simulink model "WaterRunner_closed3"  (R2013a)
settings: Solver=ode23s  StartTime=0.0  StopTime=10  RelTol=1e-3
values from neighbouring files (symbols this model uses):
  Ac = [sum(Ay), sum(Ath), sum(Aph) ... (first row only)    [SimParam_hopper.m]    (also in simParam.m = [2*sum(Ay), 2*sum(Ath))
  Cgain = 0    [searchHeightWaves.m]    (also in searchTorques.m; simParam.m = 10)
  dTorqueAmp = 1e-2    (= 0.01)    [SimParam_hopper.m]    (also in simParam.m = 0)
  dTorqueFreq = 0.5    [SimParam_hopper.m]    (also in simParam.m = 3.14159265359)
  dWaveAmp = 0    [simParam.m]
  dWaveFreq = (2*pi)/2    (= 3.14159265359)    [simParam.m]
  Filter_Coef = 1000    [SimParam_hopper.m]    (also in simParam.m)
  freq = findSSinput(y,b_water,k_water,A,Fratio,mass*g/4,w0)    [SimParam_hopper.m]    (also in findParams.m = freqs(k); simParam.m; sweepDFomega.m = FREQ(k))
  Gc = [sum(G) - mass*g ; Lx'*G ; Lz'*G]    [SimParam_hopper.m]    (also in simParam.m = [2*sum(G) - mass*g ; Lx'*G ])
  Kdf = 0.25    [SimParam_hopper.m]    (also in simParam.m = 0)
  Ke = diag([0 1])    [simParam.m]
  Mc = [mass 0 0; 0 Ix 0 ; 0 0 Iz]    [SimParam_hopper.m]    (also in simParam.m = [mass 0 ; 0 Ix])
  nullProj = eye(8) - pinvBc*Bc    [SimParam_hopper.m]    (also in simParam.m = eye(4) - pinvBc*Bc)
  omega_0 = freq*ones(8,1)    [SimParam_hopper.m]    (also in findParams.m = freq*ones(4,1); simParam.m = freq*ones(4,1); sweepDFomega.m = freq*ones(4,1))
  phase_0 = [0 pi 0 pi]    [findParams.m]    (also in simParam.m; sweepDFomega.m)
  pinvBc = pinv(Bc)    [SimParam_hopper.m]    (also in simParam.m)
  tail_density = CF_density    (= 1790)    [simParam.m]
  tail_length = 0.1    [simParam.m]
  theta = 0 *pi/180    (= 0)    [SimParam_hopper.m]    (also in simParam.m)
  y = 0.02    [SimParam_hopper.m]    (also in simParam.m = 0.015)
undefined symbols (not defined in the file or in its folder): X, Y, Z
undefined symbols (not defined in the file): cw_FL_HL, cw_FR_FL, cw_FR_HR, cw_HR_HL, FL_HL_lag, FR_FL_lag, FR_HR_lag, HR_HL_lag, K_d, K_i, K_p, phi0, tail_pad_radius, theta0, water_level, y0
libraries: nesl_utility x40, sm_lib x36, WaterRunner_lib_2 x10, dspstat3 x4, simulink x3
(part 1 of 4)
settings Model: SimulationMode=rapid-accelerator  ExtModeTrigDuration=100  Creator=nitisht  LastModifiedBy=nitisht
settings SolverCC: ZeroCrossControl=DisableAll  ZeroCrossAlgorithm=Adaptive
settings DataIOCC: SaveFinalState=on  SignalLoggingSaveFormat=ModelDataLogs  SaveOutput=off  SaveState=on  StateSaveName=tmp_raccel_xout
settings OptimizationCC: BlockReduction=off  ExpressionDepthLimit=2147483647  EfficientMapNaN2IntZero=off  SimCompilerOptimization=On
settings DebuggingCC: SolverPrmCheckMsg=none  FcnCallInpInsideContextMsg=EnableAllAsWarning
settings HardwareCC: ProdBitPerLong=64  ProdBitPerPointer=64  ProdIntDivRoundTo=Zero  ProdEndianess=LittleEndian  ProdWordSize=64  ProdHWDeviceType=Intel->x86-64  TargetBitPerLong=64  TargetBitPerPointer=64  TargetIntDivRoundTo=Zero  TargetEndianess=LittleEndian  TargetWordSize=64  TargetHWDeviceType=MATLAB Host  ProdEqTarget=off
settings RTWCC: SystemTargetFile=raccel.tlc  TemplateMakefile=raccel_default_tmf  RTWVerbose=off  ProcessScript=raccel_make_rtw_hook  RTWUseSimCustomCode=on
settings CodeAppCC: GenerateComments=off  MaxIdLength=128  MangleLength=10  SimulinkBlockComments=off
settings RaccelTargetCC: CodeReplacementLibrary=ANSI_C  ERTMultiwordTypeDef=System defined  ERTMultiwordLength=256  IsPILTarget=off  ParMdlRefBuildCompliant=off  GeneratePreprocessorConditionals=Disable all  ERTFirstTimeCompliant=off  MultiInstanceERTCode=off  EnableShiftOperators=on  ExtModeMexArgs='', 0, 36789  ENABLE_SLEXEC_SSBRIDGE=off  RTWCAPISignals=off  RTWCAPIParams=off
settings ExplorerConfigSet: InternalSimMechanicsExplorerSettings="<ExplorerConfiguration><canonicalview>default</canonicalview><TilePanel><TileInfo><Tiles Columns=\"1\" Count=\"1\" Rows=\"1\"><Column Left=\"2\" Weight=\"1\"/><Column Left=\"1126\"/><Row Top=\"2\" Weight=\"1\"/><Row Top=\"731\"/><Tile Height=\"1\" Width=\"1\" X=\"0\" Y=\"0\"/></Tiles></TileInfo><SceneInfo><SceneViewer><BGColor><R>0.60000002384185791</R><G>0.60000002384185791</G><B>0.60000002384185791</B></BGColor><Camera><Position><X>0.62960776240868022</X><Y>0.44895086159575193</Y><Z>2.4180251146380058</Z></Position><Center><X>0.10015296144366015</X><Y>-0.0072288572057211953</Y><Z>0.36408963188780596</Z></Center><Up><X>-0.10388617680904223</X><Y>0.97626280455059633</Y><Z>-0.19004893769501835</Z></Up><Left>-0.42563784714662656</Left><Right>0.42563784714662656</Right><Bottom>-0.49536256924715738</Bottom><Top>0.49536256924715738</Top></Camera></SceneViewer></SceneInfo></TilePanel></ExplorerConfiguration>"

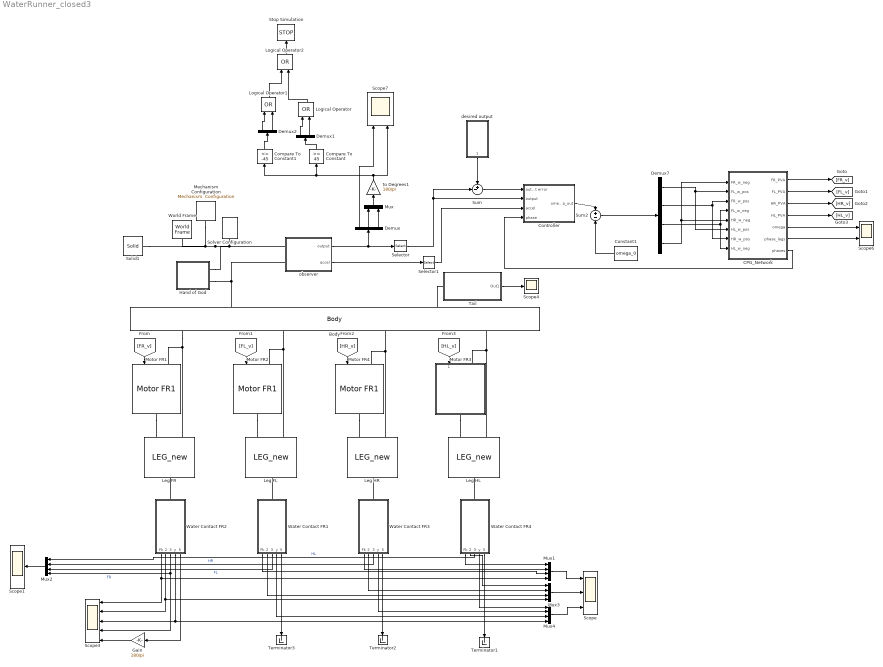
== system WaterRunner_closed3 ==
  Body : WaterRunner_lib_2/Body
  CPG_Network : Subsystem
  Compare To Constant : simulink/Logic and Bit Operations/Compare To Constant  relop=>=  const=45  OutDataTypeStr=boolean
  Compare To Constant1 : simulink/Logic and Bit Operations/Compare To Constant  relop=<=  const=-45  OutDataTypeStr=boolean
  Constant1 : Constant  Value=omega_0
  Controller : Subsystem
  Demux : Demux  Outputs=3
  Demux1 : Demux  Outputs=2
  Demux2 : Demux  Outputs=2
  Demux7 : Demux
  Gain : Gain  Gain=180/pi
  Hand of God : Subsystem
  Leg FL : WaterRunner_lib_2/LEG_new  p_L1=L1  p_L2=L2  p_L3=L3  p_L4=L4  p_L5=L5  p_CF_density=CF_density  p_bar_w=bar_w  p_bar_h=bar_h  init_pas_ang=0
  Leg FR : WaterRunner_lib_2/LEG_new  p_L1=L1  p_L2=L2  p_L3=L3  p_L4=L4  p_L5=L5  p_CF_density=CF_density  p_bar_w=bar_w  p_bar_h=bar_h  init_pas_ang=0
  Leg HL : WaterRunner_lib_2/LEG_new  p_L1=L1  p_L2=L2  p_L3=L3  p_L4=L4  p_L5=L5  p_CF_density=CF_density  p_bar_w=bar_w  p_bar_h=bar_h  init_pas_ang=0
  Leg HR : WaterRunner_lib_2/LEG_new  p_L1=L1  p_L2=L2  p_L3=L3  p_L4=L4  p_L5=L5  p_CF_density=CF_density  p_bar_w=bar_w  p_bar_h=bar_h  init_pas_ang=0
  Logical Operator : Logic  Operator=OR  AllPortsSameDT=off  OutDataTypeStr=boolean
  Logical Operator1 : Logic  Operator=OR  AllPortsSameDT=off  OutDataTypeStr=boolean
  Logical Operator2 : Logic  Operator=OR  AllPortsSameDT=off  OutDataTypeStr=boolean
  Mechanism Configuration : sm_lib/Utilities/Mechanism  Configuration  GravityVector=[0 -9.81 0]  GravityUnits=m/s^2  AllowGravitySignal=off  LinearizationDelta=0.001  BlockFunction=simmechanics.library.utilities.mechanism_configuration
  Motor FR1 : WaterRunner_lib_2/Motor FR1  init_ang=180
  Motor FR2 : WaterRunner_lib_2/Motor FR1  init_ang=0
  Motor FR3 : Subsystem  AncestorBlock=WaterRunner_lib_2/Motor FR1  mask{init_ang=-180}
      mask prompts: init_ang "Initial angle (degree)"
  Motor FR4 : WaterRunner_lib_2/Motor FR1  init_ang=0
  Mux : Mux  Inputs=2
  Mux{1..4} (4 alike) : Mux
  Scope : Scope  NumInputPorts=3
      settings: YMin=0~-2.5~-0.04  YMax=0.325~0.75~0.045
  Scope1 : Scope
      settings: ShowLegends=on  YMin=-2.5  YMax=0.75
  Scope3 : Scope  NumInputPorts=5
      settings: ShowLegends=on  YMin=0~-15~-0.125~-7.5~0  YMax=1.1~2.5~0.1~7.5~130  SaveName=ScopeData4
  Scope4 : Scope
      settings: SaveName=ScopeData2
  Scope6 : Scope  NumInputPorts=2
      settings: TimeRange=10  YMin=44~2.85  YMax=67~3.75  SaveName=cpg_omega
  Scope7 : Scope  NumInputPorts=2
      settings: TimeRange=10  YMin=-0.02~-10  YMax=0.0225~17.5  SaveName=output
  Selector : Selector  InputPortWidth=3  IndexOptions=Index vector (dialog)  Indices=[1 2]  OutputSizes=1
  Selector1 : Selector  InputPortWidth=3  IndexOptions=Index vector (dialog)  Indices=[1 2]  OutputSizes=1
  Solid1 : sm_lib/Body Elements/Solid  InertiaType=PointMass  Mass=0  MassUnits=kg  CenterOfMass=[0 0 0]  CenterOfMassUnits=m  MomentsOfInertia=[1 1 1]  MomentsOfInertiaUnits=kg*m^2  ProductsOfInertia=[0 0 0]  ProductsOfInertiaUnits=kg*m^2  DensityBased=on  Density=1000  DensityUnits=kg/(m^3)  GraphicType=FromGeometry  MarkerShape=Sphere  MarkerSize=10  MarkerSizeUnits=m  GraphicVisPropType=SimpleVisualProperties  GraphicDiffuseColor=[0.4 0.4 1.0]  GraphicSpecularColor=[0.5 0.5 0.5 1.0]  GraphicAmbientColor=[0.15 0.15 0.15 1.0]  GraphicEmissiveColor=[0.0 0.0 0.0 1.0]  GraphicShininess=75  GraphicOpacity=0.5  GeometryShape=Brick  RectangleSize=[1 1]  RectangleSizeUnits=m  BrickDimensions=[20 .001 1]  BrickDimensionUnits=m  CylinderRadius=1  CylinderRadiusUnits=m  CylinderLength=1  CylinderLengthUnits=m  SphereRadius=1  SphereRadiusUnits=m  EllipsoidRadii=[1 1 1]  EllipsoidRadiiUnits=m  ExtrusionCrossSection=[1 1; -1 1; -1 -1; 1 -1]  ExtrusionCrossSectionUnits=m  ExtrusionLength=1  ExtrusionLengthUnits=m  PolygonNumSides=3  PolygonOuterRadius=1  PolygonOuterRadiusUnits=m  ExtGeomFileUnits=m  RevolutionCrossSection=[1 1; 1 -1; 2 -1; 2 1]  RevolutionCrossSectionUnits=m  RevolutionExtent=Full  RevolutionAngle=180  RevolutionAngleUnits=deg  BlockFunction=simmechanics.library.body_elements.solid
  Solver Configuration : nesl_utility/Solver Configuration  PhysicalDomain=network_engine_domain  SubClassName=solver  LeftPortType=input  RightPortType=generic  Accelerate=off  Tones=[]  Harmonics=[]  SimulateNoise=off  Profile=off  UseLocalSampling=off  EnableSwitchedLinearOptims=on  FrequencyDomain=off  UseCCode=off  UseNewInitialization=off  DoDC=off  ResidualTolerance=1e-3  UseLocalSolver=off  LocalSolverChoice=NE_BACKWARD_EULER_ADVANCER  LocalSolverSampleTime=.001  DoFixedCost=off  MaxNonlinIter=3  MaxModeIter=2  LinearAlgebra=Sparse  DelaysMemoryBudget=1024
  Stop Simulation : Stop
  Sum : Sum  Inputs=+-|
  Sum2 : Sum  Inputs=+|-
  Tail : Subsystem
  Terminator1 : Terminator
  Terminator2 : Terminator
  Terminator3 : Terminator
  Water Contact FR1 : Subsystem
  Water Contact FR2 : Subsystem
  Water Contact FR3 : Subsystem
  Water Contact FR4 : Subsystem
  World Frame : sm_lib/Frames and  Transforms/World Frame  BlockFunction=simmechanics.library.frames_transforms.world_frame
  desired output : Subsystem
  observer : Subsystem
  to Degrees1 : Gain  Gain=180/pi
  wires:
  CPG_Network/1(FR_PVA) -> [FR_v]
  CPG_Network/2(FL_PVA) -> [FL_v]
  CPG_Network/3(HR_PVA) -> [HR_v]
  CPG_Network/4(HL_PVA) -> [HL_v]
  Mux2/1 -> Scope1/1
  Water Contact FR4/3(Vy) -> Mux2/1  "HL"
  Water Contact FR3/3(Vy) -> Mux2/2  "HR"
  Water Contact FR1/3(Vy) -> Mux2/3  "FL"
  Water Contact FR2/3(Vy) -> Scope3/4, Mux2/4  "FR"
  [FR_v] -> Motor FR1/1
  [FL_v] -> Motor FR2/1
  [HR_v] -> Motor FR4/1
  [HL_v] -> Motor FR3/1(desired speed)
  Mux1/1 -> Scope/1
  Mux3/1 -> Scope/2
  Water Contact FR4/1(Fk) -> Mux1/1
  Water Contact FR3/1(Fk) -> Mux1/2
  Water Contact FR1/1(Fk) -> Mux1/3
  Water Contact FR2/1(Fk) -> Mux1/4, Scope3/1
  Water Contact FR4/2(Fb) -> Mux3/1
  Water Contact FR3/2(Fb) -> Mux3/2
  Water Contact FR1/2(Fb) -> Mux3/3
  Water Contact FR2/2(Fb) -> Mux3/4, Scope3/2
  Mux4/1 -> Scope/3
  Water Contact FR4/4(y) -> Mux4/1
  Water Contact FR3/4(y) -> Mux4/2
  Water Contact FR1/4(y) -> Mux4/3
  Water Contact FR2/4(y) -> Mux4/4, Scope3/3
  Water Contact FR2/5(angle) -> Gain/1
  Gain/1 -> Scope3/5
  Tail/1(Out1) -> Scope4/1
  Controller/1(omega_out) -> Sum2/1
  Constant1/1 -> Sum2/2
  CPG_Network/5(omega) -> Scope6/1
  CPG_Network/6(phase_lags) -> Scope6/2
  observer/1(output) -> Demux/1, Selector/1
  Demux/2 -> Mux/1
  Demux/3 -> Mux/2
  Mux/1 -> to Degrees1/1
  to Degrees1/1 -> Compare To Constant1/1, Compare To Constant/1, Scope7/2
  Demux/1 -> Scope7/1
  desired output/1(desired output) -> Sum/1
  Water Contact FR4/5(angle) -> Terminator1/1
  Water Contact FR3/5(angle) -> Terminator2/1
  Water Contact FR1/5(angle) -> Terminator3/1
  observer/2(accel) -> Selector1/1
  Sum/1 -> Controller/1(output error)
  Sum2/1 -> Demux7/1
  Selector/1 -> Sum/2, Controller/2(output)
  Selector1/1 -> Controller/3(accel)
  Compare To Constant/1 -> Demux1/1
  Demux1/1 -> Logical Operator/1
  Demux1/2 -> Logical Operator/2
  Compare To Constant1/1 -> Demux2/1
  Demux2/1 -> Logical Operator1/1
  Demux2/2 -> Logical Operator1/2
  Logical Operator1/1 -> Logical Operator2/1
  Logical Operator/1 -> Logical Operator2/2
  Logical Operator2/1 -> Stop Simulation/1
  CPG_Network/7(phases) -> Controller/4(phase)
  Demux7/1 -> CPG_Network/6(HL_w_pos), CPG_Network/2(FL_w_pos)
  Demux7/2 -> CPG_Network/3(FR_w_pos), CPG_Network/7(HR_w_pos)
  Demux7/3 -> CPG_Network/4(FL_w_neg), CPG_Network/8(HL_w_neg)
  Demux7/4 -> CPG_Network/5(HR_w_neg), CPG_Network/1(FR_w_neg)
  connections:
  Motor FR1/RConn1 -- Leg FR/LConn1
  Body/LConn1 -- Motor FR1/LConn1 -- Leg FR/LConn2
  Water Contact FR2/LConn1 -- Leg FR/RConn1
  Leg FL/LConn2 -- Motor FR2/LConn1 -- Body/LConn2
  Motor FR2/RConn1 -- Leg FL/LConn1
  Water Contact FR1/LConn1 -- Leg FL/RConn1
  Leg HR/LConn2 -- Motor FR4/LConn1 -- Body/LConn3
  Motor FR4/RConn1 -- Leg HR/LConn1
  Water Contact FR3/LConn1 -- Leg HR/RConn1
  Motor FR3/RConn1 -- Leg HL/LConn1
  Leg HL/LConn2 -- Motor FR3/LConn1 -- Body/LConn4
  Water Contact FR4/LConn1 -- Leg HL/RConn1
  Solver Configuration/RConn1 -- Hand of God/RConn1 -- Solid1/RConn1 -- World Frame/RConn1 -- Mechanism Configuration/RConn1 -- observer/LConn1
  Tail/LConn1 -- Body/RConn2
  Body/RConn1 -- Hand of God/RConn2 -- observer/LConn2

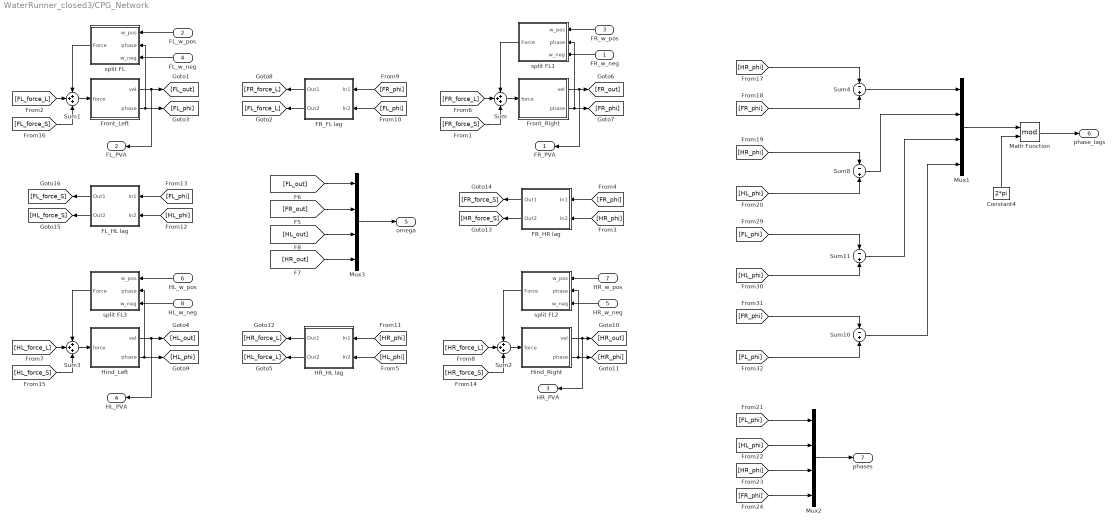
== system WaterRunner_closed3/CPG_Network ==
  FR_w_neg : Inport
  FL_w_pos : Inport  Port=2
  FR_w_pos : Inport  Port=3
  FL_w_neg : Inport  Port=4
  HR_w_neg : Inport  Port=5
  HL_w_pos : Inport  Port=6
  HR_w_pos : Inport  Port=7
  HL_w_neg : Inport  Port=8
  Constant4 : Constant  Value=2*pi
  FL_HL lag : Subsystem  mask{d_phase=FL_HL_lag, coupling_weight=cw_FL_HL}
      mask prompts: d_phase "Phase Lag"; coupling_weight "Coupling Weight"
  FR_FL lag : Subsystem  mask{d_phase=FR_FL_lag, coupling_weight=cw_FR_FL}
      mask prompts: d_phase "Phase Lag"; coupling_weight "Coupling Weight"
  FR_HR lag : Subsystem  mask{d_phase=FR_HR_lag, coupling_weight=cw_FR_HR}
      mask prompts: d_phase "Phase Lag"; coupling_weight "Coupling Weight"
  Front_Left : Subsystem  mask{init_phi=0}
      mask prompts: init_phi "Initial Phase"
  Front_Right : Subsystem  mask{init_phi=pi}
      mask prompts: init_phi "Initial Phase"
  HR_HL lag : Subsystem  mask{d_phase=HR_HL_lag, coupling_weight=cw_HR_HL}
      mask prompts: d_phase "Phase Lag"; coupling_weight "Coupling Weight"
  Hind_Left : Subsystem  mask{init_phi=pi}
      mask prompts: init_phi "Initial Phase"
  Hind_Right : Subsystem  mask{init_phi=0}
      mask prompts: init_phi "Initial Phase"
  Math Function : Math  Operator=mod  SaturateOnIntegerOverflow=on
  Mux1 : Mux
  Mux2 : Mux
  Mux3 : Mux
  Sum{,1..3} (4 alike) : Sum  Inputs=+++
  Sum{4,8,10..11} (4 alike) : Sum  Inputs=-|+
  split FL : Subsystem
  split FL1 : Subsystem
  split FL2 : Subsystem
  split FL3 : Subsystem
  FR_PVA : Outport
  FL_PVA : Outport  Port=2
  HR_PVA : Outport  Port=3
  HL_PVA : Outport  Port=4
  omega : Outport  Port=5
  phase_lags : Outport  Port=6
  phases : Outport  Port=7
  wires:
  Front_Left/2(phase) -> split FL/2(phase), [FL_phi]
  Front_Right/2(phase) -> split FL1/2(phase), [FR_phi]
  [FL_phi] -> FR_FL lag/2(In2)
  [FR_phi] -> FR_FL lag/1(In1)
  FR_FL lag/1(Out1) -> [FR_force_L]
  FR_FL lag/2(Out2) -> [FL_force_L]
  Front_Right/1(vel) -> FR_PVA/1, [FR_out]
  [FL_force_L] -> Sum1/2
  Sum1/1 -> Front_Left/1(force)
  Sum/1 -> Front_Right/1(force)
  [FR_force_L] -> Sum/2
  FR_w_pos/1 -> split FL1/1(w_pos)
  FR_w_neg/1 -> split FL1/3(w_neg)
  split FL1/1(Force) -> Sum/1
  FL_w_pos/1 -> split FL/1(w_pos)
  FL_w_neg/1 -> split FL/3(w_neg)
  Front_Left/1(vel) -> FL_PVA/1, [FL_out]
  split FL/1(Force) -> Sum1/1
  Hind_Left/2(phase) -> split FL3/2(phase), [HL_phi]
  Hind_Right/2(phase) -> [HR_phi], split FL2/2(phase)
  [HL_phi] -> HR_HL lag/2(In2)
  [HR_phi] -> HR_HL lag/1(In1)
  HR_HL lag/1(Out1) -> [HR_force_L]
  HR_HL lag/2(Out2) -> [HL_force_L]
  Hind_Right/1(vel) -> HR_PVA/1, [HR_out]
  [HL_force_L] -> Sum3/2
  Sum3/1 -> Hind_Left/1(force)
  Sum2/1 -> Hind_Right/1(force)
  [HR_force_L] -> Sum2/2
  HR_w_pos/1 -> split FL2/1(w_pos)
  HR_w_neg/1 -> split FL2/3(w_neg)
  split FL2/1(Force) -> Sum2/1
  HL_w_pos/1 -> split FL3/1(w_pos)
  HL_w_neg/1 -> split FL3/3(w_neg)
  Hind_Left/1(vel) -> HL_PVA/1, [HL_out]
  split FL3/1(Force) -> Sum3/1
  [HR_phi] -> FR_HR lag/2(In2)
  [FR_phi] -> FR_HR lag/1(In1)
  FR_HR lag/1(Out1) -> [FR_force_S]
  FR_HR lag/2(Out2) -> [HR_force_S]
  [HL_phi] -> FL_HL lag/2(In2)
  [FL_phi] -> FL_HL lag/1(In1)
  FL_HL lag/1(Out1) -> [FL_force_S]
  FL_HL lag/2(Out2) -> [HL_force_S]
  [FR_force_S] -> Sum/3
  [HR_force_S] -> Sum2/3
  [HL_force_S] -> Sum3/3
  [FL_force_S] -> Sum1/3
  Mux3/1 -> omega/1
  [FR_out] -> Mux3/2
  [FL_out] -> Mux3/1
  [HL_out] -> Mux3/3
  [HR_out] -> Mux3/4
  Sum8/1 -> Mux1/2
  [HR_phi] -> Sum8/1
  [HL_phi] -> Sum8/2
  [FL_phi] -> Sum11/1
  Sum10/1 -> Mux1/4
  [FR_phi] -> Sum10/1
  [FL_phi] -> Sum10/2
  Math Function/1 -> phase_lags/1
  Constant4/1 -> Math Function/2
  Mux1/1 -> Math Function/1
  Sum11/1 -> Mux1/3
  [HL_phi] -> Sum11/2
  Sum4/1 -> Mux1/1
  [HR_phi] -> Sum4/1
  [FR_phi] -> Sum4/2
  [FL_phi] -> Mux2/1
  [HL_phi] -> Mux2/2
  [HR_phi] -> Mux2/3
  [FR_phi] -> Mux2/4
  Mux2/1 -> phases/1

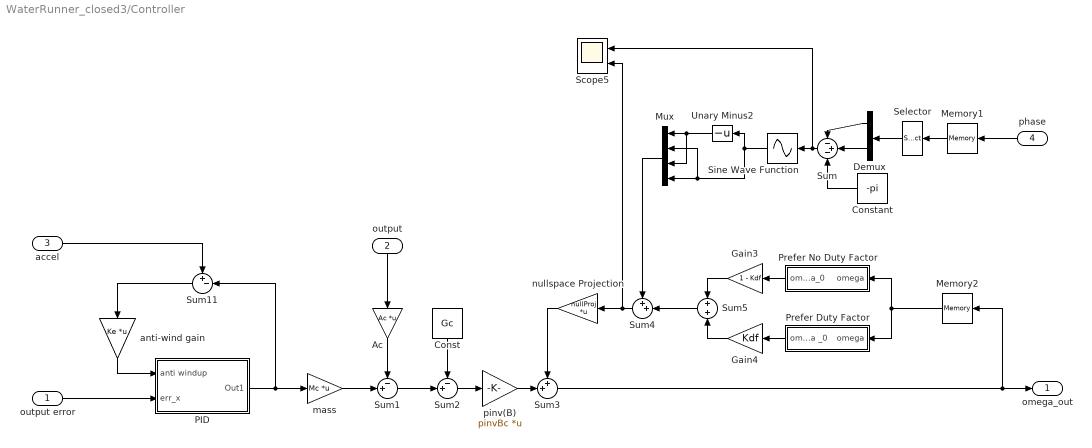
== system WaterRunner_closed3/Controller ==
  output error : Inport
  output : Inport  Port=2
  accel : Inport  Port=3
  phase : Inport  Port=4
  Ac : Gain  Gain=Ac  Multiplication=Matrix(K*u)
  Const : Constant  Value=Gc
  Constant : Constant  Value=-pi
  Demux : Demux  Outputs=2
  Gain3 : Gain  Gain=1 - Kdf
  Gain4 : Gain  Gain=Kdf
  Memory1 : Memory  X0=phase_0
  Memory2 : Memory  X0=omega_0
  Mux : Mux
  PID : Subsystem  mask{P=K_p, I=K_i, D=K_d, N=Filter_Coef}
      mask prompts: P "Proportional Gain"; I "Integral Gain"; D "Derivative Gain"; N "Filter Coefficient"
  Prefer Duty Factor : Subsystem
  Prefer No Duty Factor : Subsystem
  Scope5 : Scope  NumInputPorts=2
      settings: ShowLegends=on  TimeRange=10  YMin=-0.5~44  YMax=8~67  SaveName=command_omega
  Selector : Selector  InputPortWidth=4  IndexOptions=Index vector (dialog)  Indices=[1 4]  OutputSizes=1
  Sine Wave Function : Sin  TimeSource=Use external signal  Amplitude=Cgain  SampleTime=0
  Sum : Sum  Inputs=-+-
  Sum1 : Sum  Inputs=-+|
  Sum11 : Sum  Inputs=+-|
  Sum2 : Sum  Inputs=-+|
  Sum3 : Sum  Inputs=++|
  Sum4 : Sum  Inputs=++|
  Sum5 : Sum  Inputs=+|+
  Unary Minus2 : UnaryMinus
  anti-wind gain : Gain  Gain=Ke  Multiplication=Matrix(K*u)
  mass : Gain  Gain=Mc  Multiplication=Matrix(K*u)
  nullspace Projection : Gain  Gain=nullProj  Multiplication=Matrix(K*u)
  pinv(B) : Gain  Gain=pinvBc  Multiplication=Matrix(K*u)
  omega_out : Outport
  wires:
  output/1 -> Ac/1
  Sum2/1 -> pinv(B)/1
  mass/1 -> Sum1/2
  output error/1 -> PID/2(err_x)
  Sum3/1 -> omega_out/1, Memory2/1
  Ac/1 -> Sum1/1
  pinv(B)/1 -> Sum3/2
  nullspace Projection/1 -> Sum3/1
  Sum1/1 -> Sum2/2
  Const/1 -> Sum2/1
  PID/1(Out1) -> Sum11/2, mass/1
  accel/1 -> Sum11/1
  Sum11/1 -> anti-wind gain/1
  anti-wind gain/1 -> PID/1(anti windup)
  phase/1 -> Memory1/1
  Memory1/1 -> Selector/1
  Selector/1 -> Demux/1
  Demux/2 -> Sum/2
  Demux/1 -> Sum/1
  Sum/1 -> Scope5/1, Sine Wave Function/1
  Mux/1 -> Sum4/1
  Sum4/1 -> Scope5/2, nullspace Projection/1
  Constant/1 -> Sum/3
  Gain4/1 -> Sum5/2
  Prefer No Duty Factor/1(omega_0) -> Gain3/1
  Prefer Duty Factor/1(omega _0) -> Gain4/1
  Gain3/1 -> Sum5/1
  Memory2/1 -> Prefer Duty Factor/1(omega), Prefer No Duty Factor/1(omega)
  Sum5/1 -> Sum4/2
  Sine Wave Function/1 -> Mux/2, Mux/4, Unary Minus2/1
  Unary Minus2/1 -> Mux/3, Mux/1

== system WaterRunner_closed3/Hand of God ==
  Product : Product
  Rigid  Transform1 : sm_lib/Frames and  Transforms/Rigid  Transform  TranslationMethod=Cartesian  TranslationLengthUnit=m  TranslationStandardAxis=+Z  TranslationStandardOffset=0  TranslationCartesianOffset=[0 0 0]  TranslationROffset=0  TranslationROffsetUnits=m  TranslationZOffset=0  TranslationZOffsetUnits=m  TranslationThetaOffset=0  TranslationThetaOffsetUnits=deg  RotationMethod=AlignedAxes  RotationAngleUnits=deg  RotationStandardAxis=+Z  RotationAngle=0  RotationArbitraryAxis=[0 0 1]  FollAlignAxisA=+Y  BaseAlignAxisA=+Y  FollAlignAxisB=+Z  BaseAlignAxisB=+X  BlockFunction=simmechanics.library.frames_transforms.rigid_transform
  Rigid  Transform2 : sm_lib/Frames and  Transforms/Rigid  Transform  TranslationMethod=None  TranslationLengthUnit=m  TranslationStandardAxis=+Z  TranslationStandardOffset=0  TranslationCartesianOffset=[0 0 0]  TranslationROffset=0  TranslationROffsetUnits=m  TranslationZOffset=0  TranslationZOffsetUnits=m  TranslationThetaOffset=0  TranslationThetaOffsetUnits=deg  RotationMethod=AlignedAxes  RotationAngleUnits=deg  RotationStandardAxis=+Z  RotationAngle=0  RotationArbitraryAxis=[0 0 1]  FollAlignAxisA=+X  BaseAlignAxisA=+Z  FollAlignAxisB=+Z  BaseAlignAxisB=+Y  BlockFunction=simmechanics.library.frames_transforms.rigid_transform
  Rigid  Transform3 : sm_lib/Frames and  Transforms/Rigid  Transform  TranslationMethod=None  TranslationLengthUnit=m  TranslationStandardAxis=+Z  TranslationStandardOffset=0  TranslationCartesianOffset=[0 0 0]  TranslationROffset=0  TranslationROffsetUnits=m  TranslationZOffset=0  TranslationZOffsetUnits=m  TranslationThetaOffset=0  TranslationThetaOffsetUnits=deg  RotationMethod=AlignedAxes  RotationAngleUnits=deg  RotationStandardAxis=+Z  RotationAngle=0  RotationArbitraryAxis=[0 0 1]  FollAlignAxisA=+Y  BaseAlignAxisA=+Z  FollAlignAxisB=+X  BaseAlignAxisB=+X  BlockFunction=simmechanics.library.frames_transforms.rigid_transform
  Rigid  Transform4 : sm_lib/Frames and  Transforms/Rigid  Transform  TranslationMethod=None  TranslationLengthUnit=m  TranslationStandardAxis=+Z  TranslationStandardOffset=0  TranslationCartesianOffset=[0 0 0]  TranslationROffset=0  TranslationROffsetUnits=m  TranslationZOffset=0  TranslationZOffsetUnits=m  TranslationThetaOffset=0  TranslationThetaOffsetUnits=deg  RotationMethod=AlignedAxes  RotationAngleUnits=deg  RotationStandardAxis=+Z  RotationAngle=0  RotationArbitraryAxis=[0 0 1]  FollAlignAxisA=+Z  BaseAlignAxisA=+X  FollAlignAxisB=+Y  BaseAlignAxisB=+Y  BlockFunction=simmechanics.library.frames_transforms.rigid_transform
  Rigid  Transform5 : sm_lib/Frames and  Transforms/Rigid  Transform  TranslationMethod=None  TranslationLengthUnit=m  TranslationStandardAxis=+Z  TranslationStandardOffset=0  TranslationCartesianOffset=[0 0 0]  TranslationROffset=0  TranslationROffsetUnits=m  TranslationZOffset=0  TranslationZOffsetUnits=m  TranslationThetaOffset=0  TranslationThetaOffsetUnits=deg  RotationMethod=AlignedAxes  RotationAngleUnits=deg  RotationStandardAxis=+Z  RotationAngle=0  RotationArbitraryAxis=[0 0 1]  FollAlignAxisA=+X  BaseAlignAxisA=+Z  FollAlignAxisB=+Z  BaseAlignAxisB=+Y  BlockFunction=simmechanics.library.frames_transforms.rigid_transform
  Rigid  Transform6 : sm_lib/Frames and  Transforms/Rigid  Transform  TranslationMethod=None  TranslationLengthUnit=m  TranslationStandardAxis=+Z  TranslationStandardOffset=0  TranslationCartesianOffset=[0 0 0]  TranslationROffset=0  TranslationROffsetUnits=m  TranslationZOffset=0  TranslationZOffsetUnits=m  TranslationThetaOffset=0  TranslationThetaOffsetUnits=deg  RotationMethod=AlignedAxes  RotationAngleUnits=deg  RotationStandardAxis=+Z  RotationAngle=0  RotationArbitraryAxis=[0 0 1]  FollAlignAxisA=+Z  BaseAlignAxisA=+Y  FollAlignAxisB=+X  BaseAlignAxisB=+X  BlockFunction=simmechanics.library.frames_transforms.rigid_transform
  Scope7 : Scope
      settings: TimeRange=15  YMin=0  YMax=0.001  SaveName=command_omega2
  Simulink-PS Converter : nesl_utility/Simulink-PS Converter  PhysicalDomain=network_engine_domain  SubClassName=ps_input  LeftPortType=input  RightPortType=output  PseudoPeriodic=off  Frequencies=[]  NoiseDistribution=none  NoiseParameters=[]  Unit=1  AffineConversion=off  InputFiltering=off  SimscapeFilterOrder=1  InputFilterTimeConstant=.001  UdotUserProvided=[]
  Sine Wave : Sin  Amplitude=dTorqueAmp  Frequency=dTorqueFreq  SampleTime=0
  Step : Step  Time=3  Before=1  After=0  SampleTime=0
  Transport Delay : TransportDelay  DelayTime=2
  forward motion : sm_lib/Joints/Prismatic  Joint  SenseConstraintForceX=off  SenseConstraintForceY=off  SenseConstraintForceZ=off  SenseConstraintTorqueX=off  SenseConstraintTorqueY=off  SenseConstraintTorqueZ=off  ConstraintWrenchDir=FollowerOnBase  ConstraintWrenchFrame=BaseFrame  EquilibriumPosition=0  EquilibriumPositionUnits=m  SpringStiffness=0  SpringStiffnessUnits=N/m  DampingCoefficient=.5  DampingCoefficientUnits=N/(m/s)  ActuationMode=NoActuation  SensePosition=off  SenseVelocity=off  SenseAcceleration=off  SenseTorqueForce=off  PositionTargetValue=0  PositionTargetValueUnits=m  PositionTargetSpecify=on  PositionTargetPriority=High  VelocityTargetValue=2  VelocityTargetValueUnits=m/s  VelocityTargetSpecify=on  VelocityTargetPriority=High  BlockFunction=simmechanics.library.joints.prismatic_joint
  pitch : sm_lib/Joints/Revolute Joint  SenseConstraintForceX=off  SenseConstraintForceY=off  SenseConstraintForceZ=off  SenseConstraintTorqueX=off  SenseConstraintTorqueY=off  SenseConstraintTorqueZ=off  ConstraintWrenchDir=FollowerOnBase  ConstraintWrenchFrame=BaseFrame  EquilibriumPosition=0  EquilibriumPositionUnits=deg  SpringStiffness=0  SpringStiffnessUnits=N*m/deg  DampingCoefficient=0  DampingCoefficientUnits=N*m/(deg/s)  ActuationMode=NoActuation  SensePosition=off  SenseVelocity=off  SenseAcceleration=off  SenseTorqueForce=off  PositionTargetValue=phi0  PositionTargetValueUnits=rad  PositionTargetSpecify=on  PositionTargetPriority=High  VelocityTargetValue=0  VelocityTargetValueUnits=rad/s  VelocityTargetSpecify=on  VelocityTargetPriority=High  BlockFunction=simmechanics.library.joints.revolute_joint
  roll : sm_lib/Joints/Revolute Joint  SenseConstraintForceX=off  SenseConstraintForceY=off  SenseConstraintForceZ=off  SenseConstraintTorqueX=off  SenseConstraintTorqueY=off  SenseConstraintTorqueZ=off  ConstraintWrenchDir=FollowerOnBase  ConstraintWrenchFrame=BaseFrame  EquilibriumPosition=0  EquilibriumPositionUnits=deg  SpringStiffness=0  SpringStiffnessUnits=N*m/deg  DampingCoefficient=0  DampingCoefficientUnits=N*m/(deg/s)  ActuationMode=TorqueForceActuation  SensePosition=off  SenseVelocity=off  SenseAcceleration=off  SenseTorqueForce=off  PositionTargetValue=theta0  PositionTargetValueUnits=rad  PositionTargetSpecify=on  PositionTargetPriority=High  VelocityTargetValue=0  VelocityTargetValueUnits=rad/s  VelocityTargetSpecify=on  VelocityTargetPriority=High  BlockFunction=simmechanics.library.joints.revolute_joint
  up down : sm_lib/Joints/Prismatic  Joint  SenseConstraintForceX=off  SenseConstraintForceY=off  SenseConstraintForceZ=off  SenseConstraintTorqueX=off  SenseConstraintTorqueY=off  SenseConstraintTorqueZ=off  ConstraintWrenchDir=FollowerOnBase  ConstraintWrenchFrame=BaseFrame  EquilibriumPosition=0  EquilibriumPositionUnits=m  SpringStiffness=0  SpringStiffnessUnits=N/m  DampingCoefficient=0  DampingCoefficientUnits=N/(m/s)  ActuationMode=NoActuation  SensePosition=off  SenseVelocity=off  SenseAcceleration=off  SenseTorqueForce=off  PositionTargetValue=y0  PositionTargetValueUnits=m  PositionTargetSpecify=on  PositionTargetPriority=High  VelocityTargetValue=0  VelocityTargetValueUnits=m/s  VelocityTargetSpecify=on  VelocityTargetPriority=High  BlockFunction=simmechanics.library.joints.prismatic_joint
  Base : PMIOPort  Port=1  Side=Right
  Follower : PMIOPort  Port=2  Side=Right
  wires:
  Sine Wave/1 -> Transport Delay/1
  Transport Delay/1 -> Product/2
  Product/1 -> Scope7/1, Simulink-PS Converter/1
  Step/1 -> Product/1
  connections:
  Rigid  Transform1/LConn1 -- Base/RConn1
  Simulink-PS Converter/RConn1 -- roll/LConn2
  Rigid  Transform1/RConn1 -- forward motion/LConn1
  Rigid  Transform4/LConn1 -- pitch/RConn1
  roll/LConn1 -- Rigid  Transform4/RConn1
  forward motion/RConn1 -- Rigid  Transform2/LConn1
  pitch/LConn1 -- Rigid  Transform3/RConn1
  up down/RConn1 -- Rigid  Transform3/LConn1
  Rigid  Transform2/RConn1 -- up down/LConn1
  roll/RConn1 -- Rigid  Transform5/LConn1
  Rigid  Transform5/RConn1 -- Follower/RConn1

== system WaterRunner_closed3/Motor FR3 ==
  desired speed : Inport
  Gain2 : Gain  Gain=-1
  Memory : Memory
  PID Controller : simulink/Continuous/PID Controller  Controller=PID  TimeDomain=Continuous-time  SampleTime=1  IntegratorMethod=Forward Euler  FilterMethod=Forward Euler  Form=Parallel  P=0.001  I=0.02  D=0  N=100  InitialConditionSource=internal  InitialConditionForIntegrator=0  InitialConditionForFilter=0  ExternalReset=none  LimitOutput=off  UpperSaturationLimit=inf  LowerSaturationLimit=-inf  LinearizeAsGain=on  AntiWindupMode=none  Kb=1  TrackingMode=off  Kt=1  PParamMin=[]  PParamMax=[]  IParamMin=[]  IParamMax=[]  DParamMin=[]  DParamMax=[]  NParamMin=[]  NParamMax=[]  KbParamMin=[]  KbParamMax=[]  KtParamMin=[]  KtParamMax=[]  POutMin=[]  POutMax=[]  IOutMin=[]  IOutMax=[]  DOutMin=[]  DOutMax=[]  NOutMin=[]  NOutMax=[]  KbOutMin=[]  KbOutMax=[]  KtOutMin=[]  KtOutMax=[]  IntegratorOutMin=[]  IntegratorOutMax=[]  FilterOutMin=[]  FilterOutMax=[]  SumOutMin=[]  SumOutMax=[]  SumI1OutMin=[]  SumI1OutMax=[]  SumI2OutMin=[]  SumI2OutMax=[]  SumI3OutMin=[]  SumI3OutMax=[]  SumDOutMin=[]  SumDOutMax=[]  SaturationOutMin=[]  SaturationOutMax=[]  IntegratorContinuousStateAttributes=''  IntegratorStateMustResolveToSignalObject=off  IntegratorRTWStateStorageClass=Auto  FilterContinuousStateAttributes=''  FilterStateMustResolveToSignalObject=off  FilterRTWStateStorageClass=Auto
  Reseting : Subsystem
  Revolute Joint : sm_lib/Joints/Revolute Joint  SenseConstraintForceX=off  SenseConstraintForceY=off  SenseConstraintForceZ=off  SenseConstraintTorqueX=off  SenseConstraintTorqueY=off  SenseConstraintTorqueZ=off  ConstraintWrenchDir=FollowerOnBase  ConstraintWrenchFrame=BaseFrame  EquilibriumPosition=0  EquilibriumPositionUnits=deg  SpringStiffness=0  SpringStiffnessUnits=N*m/deg  DampingCoefficient=0.05  DampingCoefficientUnits=N*m/(deg/s)  ActuationMode=TorqueForceActuation  SensePosition=off  SenseVelocity=on  SenseAcceleration=off  SenseTorqueForce=off  PositionTargetValue=init_ang  PositionTargetValueUnits=deg  PositionTargetSpecify=on  PositionTargetPriority=High  VelocityTargetValue=-freq  VelocityTargetValueUnits=rad/s  VelocityTargetSpecify=on  VelocityTargetPriority=High  BlockFunction=simmechanics.library.joints.revolute_joint
  Saturation : Saturate  UpperLimit=300  LowerLimit=-300
  Scope : Scope  NumInputPorts=2
      settings: YMin=-67.5~-190  YMax=-42.5~0  SaveName=ScopeData4
  Sum1 : Sum  Inputs=|+-
  Sum2 : Sum  Inputs=++|
  p2 : nesl_utility/PS-Simulink Converter  PhysicalDomain=network_engine_domain  SubClassName=ps_output  LeftPortType=input  RightPortType=output  PseudoPeriodic=off  Frequencies=[]  Unit=1  AffineConversion=off
  sps : nesl_utility/Simulink-PS Converter  PhysicalDomain=network_engine_domain  SubClassName=ps_input  LeftPortType=input  RightPortType=output  PseudoPeriodic=off  Frequencies=[]  NoiseDistribution=none  NoiseParameters=[]  Unit=1  AffineConversion=off  InputFiltering=off  SimscapeFilterOrder=1  InputFilterTimeConstant=.001  UdotUserProvided=[]
  follower : PMIOPort  Port=1  Side=Right
  base : PMIOPort  Port=2  Side=Left
  wires:
  Gain2/1 -> Reseting/1(speed), Sum1/1
  p2/1 -> Scope/1, Sum1/2
  Sum2/1 -> Saturation/1
  Saturation/1 -> Memory/1
  Reseting/1(Torque) -> Sum2/1
  desired speed/1 -> Gain2/1
  Sum1/1 -> PID Controller/1
  Memory/1 -> Scope/2, sps/1
  PID Controller/1 -> Sum2/2
  connections:
  p2/LConn1 -- Revolute Joint/RConn2
  base/RConn1 -- Revolute Joint/LConn1
  Revolute Joint/RConn1 -- follower/RConn1
  sps/RConn1 -- Revolute Joint/LConn2

== system WaterRunner_closed3/Tail ==
  PassiveLink : sm_lib/Body Elements/Solid  InertiaType=CalculateFromGeometry  Mass=1  MassUnits=kg  CenterOfMass=[0 0 0]  CenterOfMassUnits=m  MomentsOfInertia=[1 1 1]  MomentsOfInertiaUnits=kg*m^2  ProductsOfInertia=[0 0 0]  ProductsOfInertiaUnits=kg*m^2  DensityBased=on  Density=tail_density*0  DensityUnits=kg/(m^3)  GraphicType=FromGeometry  MarkerShape=Sphere  MarkerSize=10  MarkerSizeUnits=m  GraphicVisPropType=SimpleVisualProperties  GraphicDiffuseColor=[0.4 1.0 0.4]  GraphicSpecularColor=[0.5 0.5 0.5 1.0]  GraphicAmbientColor=[0.15 0.15 0.15 1.0]  GraphicEmissiveColor=[0.0 0.0 0.0 1.0]  GraphicShininess=75  GraphicOpacity=1.0  GeometryShape=Brick  RectangleSize=[1 1]  RectangleSizeUnits=m  BrickDimensions=tail_dim  BrickDimensionUnits=m  CylinderRadius=1  CylinderRadiusUnits=m  CylinderLength=1  CylinderLengthUnits=m  SphereRadius=1  SphereRadiusUnits=m  EllipsoidRadii=[1 1 1]  EllipsoidRadiiUnits=m  ExtrusionCrossSection=[1 1; -1 1; -1 -1; 1 -1]  ExtrusionCrossSectionUnits=m  ExtrusionLength=1  ExtrusionLengthUnits=m  PolygonNumSides=3  PolygonOuterRadius=1  PolygonOuterRadiusUnits=m  ExtGeomFileUnits=m  RevolutionCrossSection=[1 1; 1 -1; 2 -1; 2 1]  RevolutionCrossSectionUnits=m  RevolutionExtent=Full  RevolutionAngle=180  RevolutionAngleUnits=deg  BlockFunction=simmechanics.library.body_elements.solid
  Solid : sm_lib/Body Elements/Solid  InertiaType=PointMass  Mass=0  MassUnits=kg  CenterOfMass=[0 0 0]  CenterOfMassUnits=m  MomentsOfInertia=[1 1 1]  MomentsOfInertiaUnits=kg*m^2  ProductsOfInertia=[0 0 0]  ProductsOfInertiaUnits=kg*m^2  DensityBased=on  Density=0  DensityUnits=kg/(m^3)  GraphicType=FromGeometry  MarkerShape=Sphere  MarkerSize=10  MarkerSizeUnits=m  GraphicVisPropType=SimpleVisualProperties  GraphicDiffuseColor=[0.5 0.5 0.5]  GraphicSpecularColor=[0.5 0.5 0.5 1.0]  GraphicAmbientColor=[0.15 0.15 0.15 1.0]  GraphicEmissiveColor=[0.0 0.0 0.0 1.0]  GraphicShininess=75  GraphicOpacity=1.0  GeometryShape=Cylinder  RectangleSize=[1 1]  RectangleSizeUnits=m  BrickDimensions=[1 1 1]  BrickDimensionUnits=m  CylinderRadius=tail_pad_radius  CylinderRadiusUnits=m  CylinderLength=0.001  CylinderLengthUnits=m  SphereRadius=1  SphereRadiusUnits=m  EllipsoidRadii=[1 1 1]  EllipsoidRadiiUnits=m  ExtrusionCrossSection=[1 1; -1 1; -1 -1; 1 -1]  ExtrusionCrossSectionUnits=m  ExtrusionLength=1  ExtrusionLengthUnits=m  PolygonNumSides=3  PolygonOuterRadius=1  PolygonOuterRadiusUnits=m  ExtGeomFileUnits=m  RevolutionCrossSection=[1 1; 1 -1; 2 -1; 2 1]  RevolutionCrossSectionUnits=m  RevolutionExtent=Full  RevolutionAngle=180  RevolutionAngleUnits=deg  BlockFunction=simmechanics.library.body_elements.solid
  Water Contact HR1 : Subsystem
  pad tran : sm_lib/Frames and  Transforms/Rigid  Transform  TranslationMethod=StandardAxis  TranslationLengthUnit=m  TranslationStandardAxis=-Y  TranslationStandardOffset=0.0015  TranslationCartesianOffset=[0 0 0.25]  TranslationROffset=0  TranslationROffsetUnits=m  TranslationZOffset=0  TranslationZOffsetUnits=m  TranslationThetaOffset=0  TranslationThetaOffsetUnits=deg  RotationMethod=AlignedAxes  RotationAngleUnits=deg  RotationStandardAxis=+Z  RotationAngle=0  RotationArbitraryAxis=[0 0 1]  FollAlignAxisA=+X  BaseAlignAxisA=+X  FollAlignAxisB=+Y  BaseAlignAxisB=+Z  BlockFunction=simmechanics.library.frames_transforms.rigid_transform
  tail_tr_1 : sm_lib/Frames and  Transforms/Rigid  Transform  TranslationMethod=None  TranslationLengthUnit=m  TranslationStandardAxis=+Z  TranslationStandardOffset=0  TranslationCartesianOffset=[0 0 0]  TranslationROffset=0  TranslationROffsetUnits=m  TranslationZOffset=0  TranslationZOffsetUnits=m  TranslationThetaOffset=0  TranslationThetaOffsetUnits=deg  RotationMethod=StandardAxis  RotationAngleUnits=deg  RotationStandardAxis=+Z  RotationAngle=tail_angle  RotationArbitraryAxis=[0 0 1]  FollAlignAxisA=+X  BaseAlignAxisA=+Y  FollAlignAxisB=+Y  BaseAlignAxisB=+Z  BlockFunction=simmechanics.library.frames_transforms.rigid_transform
  tail_tr_2 : sm_lib/Frames and  Transforms/Rigid  Transform  TranslationMethod=StandardAxis  TranslationLengthUnit=m  TranslationStandardAxis=-X  TranslationStandardOffset=tail_length/2  TranslationCartesianOffset=[0 0 0]  TranslationROffset=0  TranslationROffsetUnits=m  TranslationZOffset=0  TranslationZOffsetUnits=m  TranslationThetaOffset=0  TranslationThetaOffsetUnits=deg  RotationMethod=None  RotationAngleUnits=deg  RotationStandardAxis=+Z  RotationAngle=0  RotationArbitraryAxis=[0 0 1]  FollAlignAxisA=+X  BaseAlignAxisA=+Y  FollAlignAxisB=+Y  BaseAlignAxisB=+Z  BlockFunction=simmechanics.library.frames_transforms.rigid_transform
  tail_tr_3 : sm_lib/Frames and  Transforms/Rigid  Transform  TranslationMethod=StandardAxis  TranslationLengthUnit=m  TranslationStandardAxis=-X  TranslationStandardOffset=tail_length/2  TranslationCartesianOffset=[0 0 0]  TranslationROffset=0  TranslationROffsetUnits=m  TranslationZOffset=0  TranslationZOffsetUnits=m  TranslationThetaOffset=0  TranslationThetaOffsetUnits=deg  RotationMethod=None  RotationAngleUnits=deg  RotationStandardAxis=+Z  RotationAngle=0  RotationArbitraryAxis=[0 0 1]  FollAlignAxisA=+X  BaseAlignAxisA=+Y  FollAlignAxisB=+Y  BaseAlignAxisB=+Z  BlockFunction=simmechanics.library.frames_transforms.rigid_transform
  Conn1 : PMIOPort  Port=1  Side=Left
  Out1 : Outport
  wires:
  Water Contact HR1/1(Fb) -> Out1/1
  connections:
  tail_tr_2/LConn1 -- tail_tr_1/RConn1
  tail_tr_2/RConn1 -- PassiveLink/RConn1 -- tail_tr_3/LConn1
  tail_tr_3/RConn1 -- Water Contact HR1/LConn1 -- pad tran/LConn1
  tail_tr_1/LConn1 -- Conn1/RConn1
  pad tran/RConn1 -- Solid/RConn1

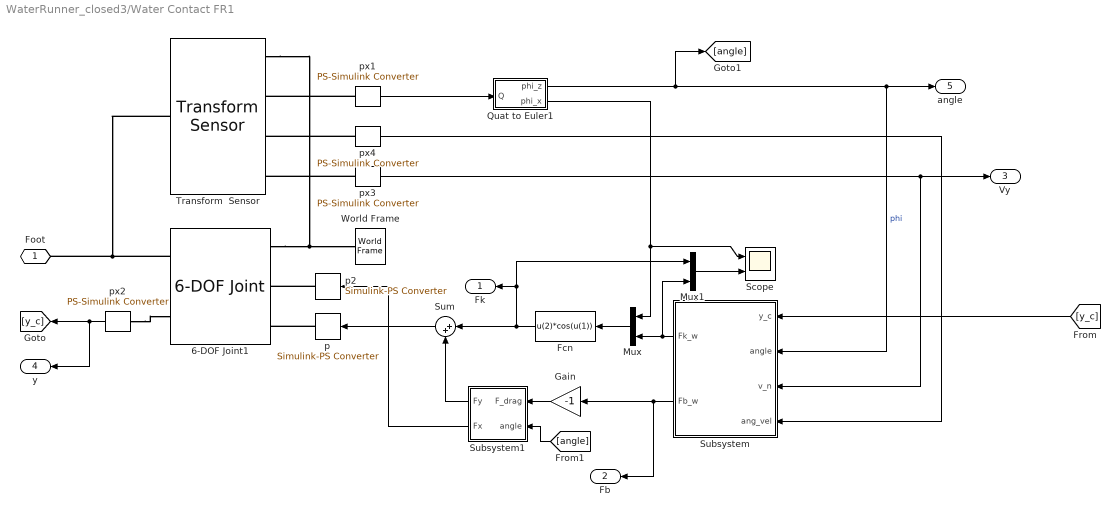
== system WaterRunner_closed3/Water Contact FR1 ==
  6-DOF Joint1 : sm_lib/Joints/6-DOF Joint  SenseConstraintForceX=off  SenseConstraintForceY=off  SenseConstraintForceZ=off  SenseConstraintTorqueX=off  SenseConstraintTorqueY=off  SenseConstraintTorqueZ=off  ConstraintWrenchDir=FollowerOnBase  ConstraintWrenchFrame=BaseFrame  PxEquilibriumPosition=0  PxEquilibriumPositionUnits=m  PxSpringStiffness=0  PxSpringStiffnessUnits=N/m  PxDampingCoefficient=0  PxDampingCoefficientUnits=N/(m/s)  PxActuationMode=TorqueForceActuation  PxSensePosition=off  PxSenseVelocity=off  PxSenseAcceleration=off  PxSenseTorqueForce=off  PxPositionTargetValue=0  PxPositionTargetValueUnits=m  PxPositionTargetSpecify=off  PxPositionTargetPriority=High  PxVelocityTargetValue=0  PxVelocityTargetValueUnits=m/s  PxVelocityTargetSpecify=off  PxVelocityTargetPriority=High  PyEquilibriumPosition=0  PyEquilibriumPositionUnits=m  PySpringStiffness=0  PySpringStiffnessUnits=N/m  PyDampingCoefficient=0  PyDampingCoefficientUnits=N/(m/s)  PyActuationMode=TorqueForceActuation  PySensePosition=on  PySenseVelocity=off  PySenseAcceleration=off  PySenseTorqueForce=off  PyPositionTargetValue=0  PyPositionTargetValueUnits=m  PyPositionTargetSpecify=off  PyPositionTargetPriority=High  PyVelocityTargetValue=0  PyVelocityTargetValueUnits=m/s  PyVelocityTargetSpecify=off  PyVelocityTargetPriority=High  PzEquilibriumPosition=0  PzEquilibriumPositionUnits=m  PzSpringStiffness=0  PzSpringStiffnessUnits=N/m  PzDampingCoefficient=0  PzDampingCoefficientUnits=N/(m/s)  PzActuationMode=NoActuation  PzSensePosition=off  PzSenseVelocity=off  PzSenseAcceleration=off  PzSenseTorqueForce=off  PzPositionTargetValue=0  PzPositionTargetValueUnits=m  PzPositionTargetSpecify=off  PzPositionTargetPriority=High  PzVelocityTargetValue=0  PzVelocityTargetValueUnits=m/s  PzVelocityTargetSpecify=off  PzVelocityTargetPriority=High  SphDefPosRotationMethod=None  SphDefPosRotationAngleUnits=deg  SphDefPosRotationStandardAxis=+Z  SphDefPosRotationAngle=0  SphDefPosRotationArbitraryAxis=[0 0 1]  SphDefPosFollAlignAxisA=+X  SphDefPosBaseAlignAxisA=+Y  SphDefPosFollAlignAxisB=+Y  SphDefPosBaseAlignAxisB=+Z  SphEqPosRotationMethod=None  SphEqPosRotationAngleUnits=deg  SphEqPosRotationStandardAxis=+Z  SphEqPosRotationAngle=0  SphEqPosRotationArbitraryAxis=[0 0 1]  SphEqPosFollAlignAxisA=+X  SphEqPosBaseAlignAxisA=+Y  SphEqPosFollAlignAxisB=+Y  SphEqPosBaseAlignAxisB=+Z  SphSpringStiffness=0  SphSpringStiffnessUnits=N*m/deg  SphDampingCoefficient=0  SphDampingCoefficientUnits=N*m/(deg/s)  SphActuateTorqueX=off  SphActuateTorqueY=off  SphActuateTorqueZ=off  SphActuateTorque=off  SphActuationMode=NoActuation  SphActuationFrame=BaseFrame  SphSensePosition=off  SphSenseVelocityX=off  SphSenseVelocityY=off  SphSenseVelocityZ=off  SphSenseVelocity=off  SphSenseAccelerationX=off  SphSenseAccelerationY=off  SphSenseAccelerationZ=off  SphSenseAcceleration=off  SphSenseTorqueX=off  SphSenseTorqueY=off  SphSenseTorqueZ=off  SphSenseTorqueForce=off  SphSensingFrame=BaseFrame  SphPositionTargetRotationMethod=None  SphPositionTargetRotationAngleUnits=deg  SphPositionTargetRotationStandardAxis=+Z  SphPositionTargetRotationAngle=0  SphPositionTargetRotationArbitraryAxis=[0 0 1]  SphPositionTargetFollAlignAxisA=+X  SphPositionTargetBaseAlignAxisA=+Y  SphPositionTargetFollAlignAxisB=+Y  SphPositionTargetBaseAlignAxisB=+Z  SphPositionTargetSpecify=off  SphPositionTargetPriority=High  SphVelocityTargetValue=[0 0 0]  SphVelocityTargetValueUnits=deg/s  SphVelocityTargetSpecify=off  SphVelocityTargetPriority=High  SphVelocityTargetInFollowerFrame=on  BlockFunction=simmechanics.library.joints.sixdof_joint
  Fcn : Fcn  Expr=u(2)*cos(u(1))
  Gain : Gain  Gain=-1
  Mux : Mux  Inputs=2
  Mux1 : Mux  Inputs=2
  Quat to Euler1 : Subsystem
  Scope : Scope  NumInputPorts=2
      settings: YMin=-0.19~0  YMax=0.04~0.7  SaveName=ScopeData3
  Subsystem : Subsystem
  Subsystem1 : Subsystem
  Sum : Sum  Inputs=|++
  Transform  Sensor : sm_lib/Frames and  Transforms/Transform  Sensor  MeasurementFrame=NonRotatingBase  SenseAngle=off  SenseAxis=off  SenseAngle1=off  SenseAngle2=off  SenseAngle3=off  SenseQ=on  SenseR=off  SenseOmegaX=off  SenseOmegaY=off  SenseOmegaZ=on  SenseOmega1=off  SenseOmega2=off  SenseOmega3=off  SenseQDot=off  SenseRDot=off  SenseAlphaX=off  SenseAlphaY=off  SenseAlphaZ=off  SenseAlpha1=off  SenseAlpha2=off  SenseAlpha3=off  SenseQDDot=off  SenseRDDot=off  SenseX=off  SenseY=off  SenseZ=off  SenseRad=off  SenseAzim=off  SenseDist=off  SenseInc=off  SenseXDot=off  SenseYDot=on  SenseZDot=off  SenseRadDot=off  SenseAzimDot=off  SenseDistDot=off  SenseIncDot=off  SenseXDDot=off  SenseYDDot=off  SenseZDDot=off  SenseRadDDot=off  SenseAzimDDot=off  SenseDistDDot=off  SenseIncDDot=off  BlockFunction=simmechanics.library.frames_transforms.transform_sensor
  World Frame : sm_lib/Frames and  Transforms/World Frame  BlockFunction=simmechanics.library.frames_transforms.world_frame
  p : nesl_utility/Simulink-PS Converter  PhysicalDomain=network_engine_domain  SubClassName=ps_input  LeftPortType=input  RightPortType=output  PseudoPeriodic=off  Frequencies=[]  NoiseDistribution=none  NoiseParameters=[]  Unit=1  AffineConversion=off  InputFiltering=off  SimscapeFilterOrder=1  InputFilterTimeConstant=.001  UdotUserProvided=[]
  p2 : nesl_utility/Simulink-PS Converter  PhysicalDomain=network_engine_domain  SubClassName=ps_input  LeftPortType=input  RightPortType=output  PseudoPeriodic=off  Frequencies=[]  NoiseDistribution=none  NoiseParameters=[]  Unit=1  AffineConversion=off  InputFiltering=off  SimscapeFilterOrder=1  InputFilterTimeConstant=.001  UdotUserProvided=[]
  px{1..4} (4 alike) : nesl_utility/PS-Simulink Converter  PhysicalDomain=network_engine_domain  SubClassName=ps_output  LeftPortType=input  RightPortType=output  PseudoPeriodic=off  Frequencies=[]  Unit=1  AffineConversion=off
  Foot : PMIOPort  Port=1  Side=Left
  Fk : Outport
  Fb : Outport  Port=2
  Vy : Outport  Port=3
  y : Outport  Port=4
  angle : Outport  Port=5
  wires:
  Subsystem/2(Fb_w) -> Gain/1, Fb/1
  px3/1 -> Vy/1, Subsystem/3(v_n)
  Quat to Euler1/1(phi_z) -> [angle], Subsystem/2(angle), angle/1  "phi"
  px1/1 -> Quat to Euler1/1(Q)
  px4/1 -> Subsystem/4(ang_vel)
  px2/1 -> [y_c], y/1
  [angle] -> Subsystem1/2(angle)
  Sum/1 -> p/1
  Subsystem1/1(Fy) -> Sum/2
  Gain/1 -> Subsystem1/1(F_drag)
  Subsystem1/2(Fx) -> p2/1
  Subsystem/1(Fk_w) -> Mux1/2, Mux/2
  Mux/1 -> Fcn/1
  Fcn/1 -> Mux1/1, Fk/1, Sum/1
  Quat to Euler1/2(phi_x) -> Mux/1, Scope/1
  Mux1/1 -> Scope/2
  [y_c] -> Subsystem/1(y_c)
  connections:
  Transform  Sensor/RConn1 -- World Frame/RConn1 -- 6-DOF Joint1/LConn1
  Transform  Sensor/LConn1 -- Foot/RConn1 -- 6-DOF Joint1/RConn1
  px2/LConn1 -- 6-DOF Joint1/RConn2
  p/RConn1 -- 6-DOF Joint1/LConn3
  px1/LConn1 -- Transform  Sensor/RConn2
  p2/RConn1 -- 6-DOF Joint1/LConn2
  px3/LConn1 -- Transform  Sensor/RConn4
  px4/LConn1 -- Transform  Sensor/RConn3
